simulink model "pwm2_PIDU_task"  (Simulink 3.00)
libraries: mathlib x2, execlib x1, reglib x1, arclib x1

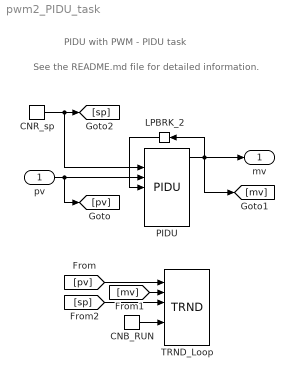
== system pwm2_PIDU_task ==
  note: See the README.md file for detailed information.
  note: PIDU with PWM - PIDU task
  pv : Inport  Port=1
  CNB_RUN : mathlib/CNB  YCN=on
  CNR_sp : mathlib/CNR  ycn=0
  LPBRK_2 : execlib/LPBRK  Orientation=left
  PIDU : reglib/PIDU  irtype=7: PID  RACT=off  k=0.1  ti=10  td=2.5  nd=4  b=1  c=0  tt=1  hilim=1  lolim=-1  dz=0  icotype=1: Analog
  TRND_Loop : arclib/TRND  n=3  l=100  btype=8  ptype1=1: Store  ptype2=1: Store  ptype3=1: Store  ptype4=1: Store  pfac=1  afac=0  arc=0  id=1  Title=Trend Title  timesrc=1
  mv : Outport  Port=1
  wires:
  CNB_RUN/1 -> TRND_Loop/5
  CNR_sp/1 -> [sp], PIDU/2
  [pv] -> TRND_Loop/1
  [mv] -> TRND_Loop/2
  [sp] -> TRND_Loop/3
  LPBRK_2/1 -> PIDU/4
  PIDU/1 -> [mv], LPBRK_2/1, mv/1
  pv/1 -> [pv], PIDU/3
